simulink library "dsppolyfun"  (Simulink 8.0)
settings: Solver=ode45  SolverMode=SingleTasking  StartTime=0.0  StopTime=10.0  RelTol=1e-3
values from neighbouring files (symbols this model uses):
  D = D + B    [rebuffer_delay.m]
  V = Wt - Wopt    [msesim.m]    (also in rebuffer_delay.m = 0)
libraries: dspsigattribs x3, dspsolvers x1
settings Model: RequirementInfo=9  Creator=sconahan  LastModifiedBy=lij  CovMetricSettings=d  ExtModeAutoUpdateStatusClock=off

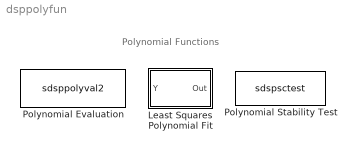
== system dsppolyfun ==
  note: Polynomial Functions
  Least Squares Polynomial Fit : Subsystem  mask(Least Squares Polynomial Fit){X=(0:31) / 31, N=3}
      mask prompts: X "Control points (X):"; N "Polynomial order (N):"
      mask help: Find the coefficients of a polynomial P(X) of order N that fits the input data U, such that P(X) best approximates U in a least-squares sense. The input vector U must have the same length as X.
      mask init:
      | % construct Vandermonde matrix
      | X=double(X(:));
      | N=double(N(1));
      | V(:,N+1) = ones(length(X),1); V(:,N) = X;
      | for j = N-1:-1:1, V(:,j) = X.*V(:,j+1); end
      mask Help: eval('blocksethelp');
      mask Display: disp('Polyfit')
  Polynomial Evaluation : S-Function  FunctionName=sdsppolyval2  Parameters=constCoeffs,useConstCoeffs  EnableBusSupport=off  mask(Polynomial Evaluation){useConstCoeffs=off, constCoeffs=[5 4 3 2 1]}
      mask prompts: useConstCoeffs "Use constant coefficients"; constCoeffs "Constant coefficients:"
      mask help:
      | Apply specified polynomial function to input.
      |
      | Example: [1 3 5] represents u^2 + 3u + 5.
      mask init:
      | [p,xy] = dspblkpolyval('icon');
      mask Help: eval('blocksethelp');
      mask CallbackString: dspblkpolyval|
      mask Display:
      | port_label(p.in1,   p.i1,  p.i1s);
      | port_label(p.in2,   p.i2,  p.i2s);
      | port_label(p.out, p.o1, p.o1s);
      | disp('Polyval')
  Polynomial Stability Test : S-Function  FunctionName=sdspsctest  EnableBusSupport=off
      mask Type: Polynomial Stability Test
      mask Description: Determines if all roots of the input polynomial lie inside the unit circle.  Implemented using the Schur-Cohn algorithm.
      mask Help: eval('blocksethelp');
      mask Display: disp('|roots(u)| < 1')

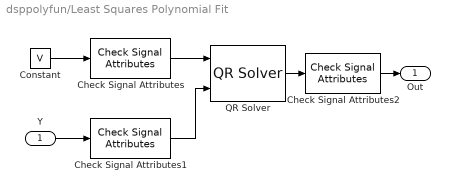
== system dsppolyfun/Least Squares Polynomial Fit ==
  Y : Inport
  Check Signal Attributes : dspsigattribs/Check Signal Attributes  SystemSampleTime=-1  SigAttribCheckMethod=Does not match attributes exactly  Complexity=Ignore  Frame=Ignore  DimsCheckMethod=Ignore  Dimensions=1-D  DatatypeCheckMethod=Is...  DatatypeGeneral=Floating-point  DtypeFloatSpecific=Any floating-point  DtypeFixedSpecific=Any fixed-point  DtypeIntSpecific=Any integer  SampleMode=Ignore
  Check Signal Attributes1 : dspsigattribs/Check Signal Attributes  SystemSampleTime=-1  SigAttribCheckMethod=Does not match attributes exactly  Complexity=Ignore  Frame=Ignore  DimsCheckMethod=Ignore  Dimensions=1-D  DatatypeCheckMethod=Is...  DatatypeGeneral=Floating-point  DtypeFloatSpecific=Any floating-point  DtypeFixedSpecific=Any fixed-point  DtypeIntSpecific=Any integer  SampleMode=Ignore
  Check Signal Attributes2 : dspsigattribs/Check Signal Attributes  SystemSampleTime=-1  SigAttribCheckMethod=Does not match attributes exactly  Complexity=Ignore  Frame=Ignore  DimsCheckMethod=Ignore  Dimensions=1-D  DatatypeCheckMethod=Is...  DatatypeGeneral=Floating-point  DtypeFloatSpecific=Any floating-point  DtypeFixedSpecific=Any fixed-point  DtypeIntSpecific=Any integer  SampleMode=Ignore
  Constant : Constant  Value=V  OutDataTypeStr=Inherit: Inherit via back propagation
  QR Solver : dspsolvers/QR Solver
  Out : Outport
  wires:
  Y/1 -> Check Signal Attributes1/1
  QR Solver/1 -> Check Signal Attributes2/1
  Constant/1 -> Check Signal Attributes/1
  Check Signal Attributes/1 -> QR Solver/1
  Check Signal Attributes1/1 -> QR Solver/2
  Check Signal Attributes2/1 -> Out/1
